simulink model "simple_test_rchg_simulink"  (Simulink 7.8)
settings: Solver=VariableStepDiscrete  StartTime=0.0  StopTime=10.0  RelTol=1e-3
values from neighbouring files (symbols this model uses):
  r_dt = vmodel_config.sample_time    [single_clock_pr_test.m]
settings Model: Creator=chuh  LastModifiedBy=chuh

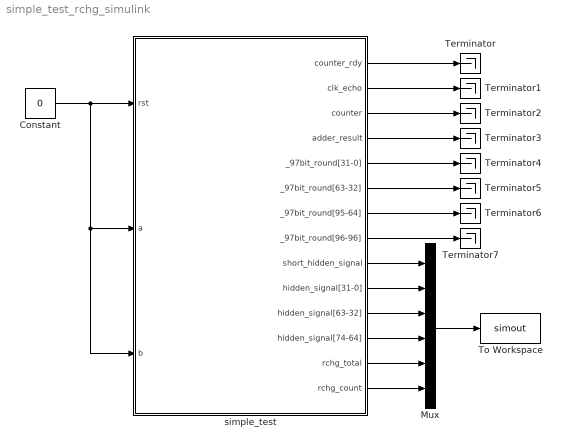
== system simple_test_rchg_simulink ==
  Constant : Constant  Value=0
  Mux : Mux  Inputs=6
  Terminator{,1..7} (8 alike) : Terminator
  To Workspace : ToWorkspace  VariableName=simout  SampleTime=r_dt  SaveFormat=Array
  simple_test : Subsystem  mask(simple_test){params_samples=r_dt, params_freq=1}
      mask prompts: params_samples "Sample time:"; params_freq "FPGA frequency (MHz):"
      mask help:
      | input rst
      | input a[30:0]
      | input b[30:0]
      | output counter_rdy
      | output clk_echo
      | output counter[15:0]
      | output adder_result[31:0]
      | output _97bit_round[96:0]
      | output short_hidden_signal[12:0]
      | output hidden_signal[74:0]
      | output rchg_total[31:0]
      | output rchg_count[31:0]
      mask Help:
      | input rst
      | input a[30:0]
      | input b[30:0]
      | output counter_rdy
      | output clk_echo
      | output counter[15:0]
      | output adder_result[31:0]
      | output _97bit_round[96:0]
      | output short_hidden_signal[12:0]
      | output hidden_signal[74:0]
      | output rchg_total[31:0]
      | output rchg_count[31:0]
  wires:
  simple_test/1(counter_rdy) -> Terminator/1
  simple_test/2(clk_echo) -> Terminator1/1
  simple_test/3(counter) -> Terminator2/1
  simple_test/4(adder_result) -> Terminator3/1
  simple_test/5(_97bit_round[31-0]) -> Terminator4/1
  simple_test/6(_97bit_round[63-32]) -> Terminator5/1
  simple_test/7(_97bit_round[95-64]) -> Terminator6/1
  simple_test/8(_97bit_round[96-96]) -> Terminator7/1
  Constant/1 -> simple_test/1(rst), simple_test/2(a), simple_test/3(b)
  simple_test/9(short_hidden_signal) -> Mux/1
  simple_test/10(hidden_signal[31-0]) -> Mux/2
  simple_test/11(hidden_signal[63-32]) -> Mux/3
  simple_test/12(hidden_signal[74-64]) -> Mux/4
  simple_test/13(rchg_total) -> Mux/5
  simple_test/14(rchg_count) -> Mux/6
  Mux/1 -> To Workspace/1

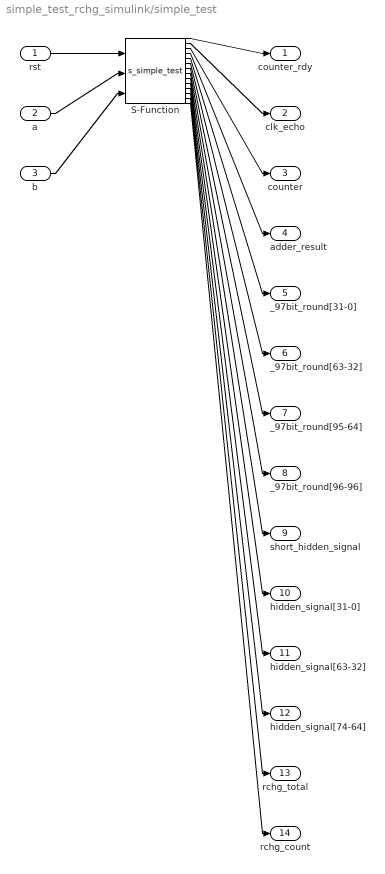
== system simple_test_rchg_simulink/simple_test ==
  rst : Inport  OutDataTypeStr=double  SampleTime=5e-07
  a : Inport  Port=2  OutDataTypeStr=double  SampleTime=5e-07
  b : Inport  Port=3  OutDataTypeStr=double  SampleTime=5e-07
  S-Function : S-Function  FunctionName=s_simple_test  Parameters=params_samples, params_freq  EnableBusSupport=off
  counter_rdy : Outport  OutDataTypeStr=uint32  SampleTime=5e-07
  clk_echo : Outport  Port=2  OutDataTypeStr=uint32  SampleTime=5e-07
  counter : Outport  Port=3  OutDataTypeStr=uint32  SampleTime=5e-07
  adder_result : Outport  Port=4  OutDataTypeStr=uint32  SampleTime=5e-07
  _97bit_round[31-0] : Outport  Port=5  OutDataTypeStr=uint32  SampleTime=5e-07
  _97bit_round[63-32] : Outport  Port=6  OutDataTypeStr=uint32  SampleTime=5e-07
  _97bit_round[95-64] : Outport  Port=7  OutDataTypeStr=uint32  SampleTime=5e-07
  _97bit_round[96-96] : Outport  Port=8  OutDataTypeStr=uint32  SampleTime=5e-07
  short_hidden_signal : Outport  Port=9  OutDataTypeStr=uint32  SampleTime=5e-07
  hidden_signal[31-0] : Outport  Port=10  OutDataTypeStr=uint32  SampleTime=5e-07
  hidden_signal[63-32] : Outport  Port=11  OutDataTypeStr=uint32  SampleTime=5e-07
  hidden_signal[74-64] : Outport  Port=12  OutDataTypeStr=uint32  SampleTime=5e-07
  rchg_total : Outport  Port=13  OutDataTypeStr=uint32  SampleTime=5e-07
  rchg_count : Outport  Port=14  OutDataTypeStr=uint32  SampleTime=5e-07
  wires:
  rst/1 -> S-Function/1
  a/1 -> S-Function/2
  b/1 -> S-Function/3
  S-Function/1 -> counter_rdy/1
  S-Function/2 -> clk_echo/1
  S-Function/3 -> counter/1
  S-Function/4 -> adder_result/1
  S-Function/5 -> _97bit_round[31-0]/1
  S-Function/6 -> _97bit_round[63-32]/1
  S-Function/7 -> _97bit_round[95-64]/1
  S-Function/8 -> _97bit_round[96-96]/1
  S-Function/9 -> short_hidden_signal/1
  S-Function/10 -> hidden_signal[31-0]/1
  S-Function/11 -> hidden_signal[63-32]/1
  S-Function/12 -> hidden_signal[74-64]/1
  S-Function/13 -> rchg_total/1
  S-Function/14 -> rchg_count/1
